simulink model "simu"  (R2023a)
settings: Solver=FixedStepAuto  StartTime=0.0  StopTime=10  RelTol=1e-3
undefined symbols (not defined in the file): Kalpha, Kbeta, Krho, theta_0, x_0, y_0
settings Model: Creator=daneydem1u  LastModifiedBy=daneydem1u

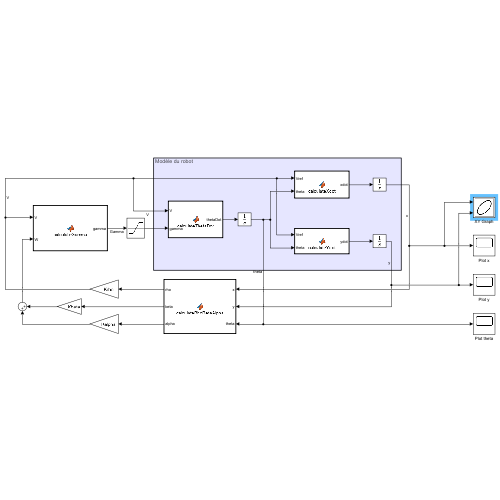
[thumbnail: Simulink's stored preview of the top-level diagram]
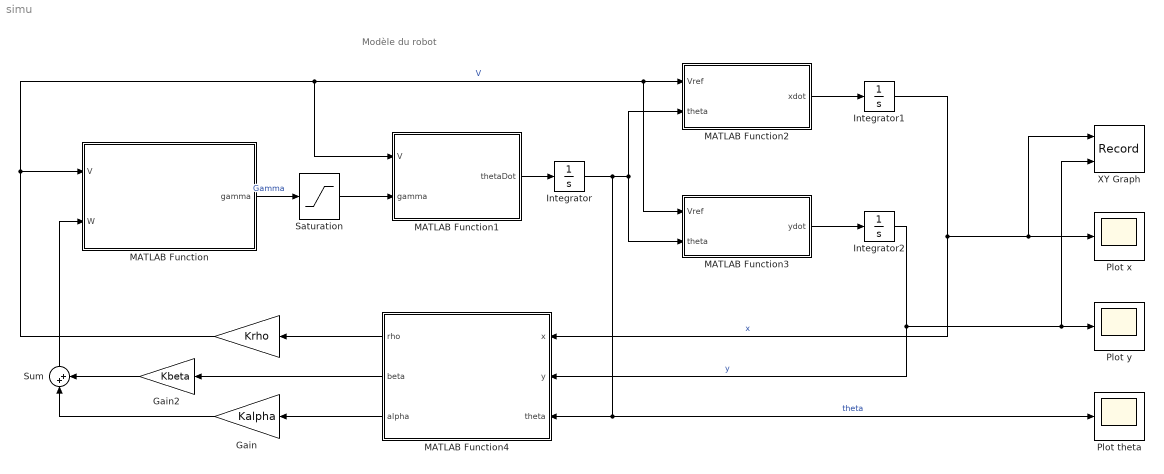
== system simu ==
  note: Modèle du robot
  " " : Gain  Gain=Krho
  Gain : Gain  Gain=Kalpha
  Gain2 : Gain  Gain=Kbeta
  Integrator : Integrator  InitialCondition=theta_0
  Integrator1 : Integrator  InitialCondition=x_0
  Integrator2 : Integrator  InitialCondition=y_0
  MATLAB Function : MATLAB Function  TreatAsAtomicUnit=on
  MATLAB Function1 : MATLAB Function  TreatAsAtomicUnit=on
  MATLAB Function2 : MATLAB Function  TreatAsAtomicUnit=on
  MATLAB Function3 : MATLAB Function  TreatAsAtomicUnit=on
  MATLAB Function4 : MATLAB Function  TreatAsAtomicUnit=on
  Plot theta : Scope
  Plot x : Scope
  Plot y : Scope
  Saturation : Saturate  UpperLimit=pi/2  LowerLimit=-pi/2
  Sum : Sum  Inputs=|++
  XY Graph : Record  FileSettingsInternal="{\"entries\":[{\"content\":{\"excelSettings\":{\"content\":{},\"type\":\"Streamout.ExcelSettings\"}},\"type\":\"Streamout.FileSettingStorage\",\"uuid\":\"87b38950-ab84-4d4e-b85e-4042bda6b861\"}],\"packageUris\":[\"http://schema.mathworks.com/mf0/streamout_blocks/R2020a\"],\"version\":\"1.0\"}"  Layout=[1 1]  SignalsInternal="{\"entries\":[{\"content\":{\"signals\":[{\"content\":{\"blockPath\":[\"simu/XY Graph\"],\"dimensions\":[1],\"domain\":\"simu/XY Graph\",\"lineColor\":\"#a2142f\",\"plots\":[1],\"port\":1,\"sid\":[\"\"],\"signalID\":212,\"signalName\":\"x\"},\"type\":\"RecordBlkView.Signal\",\"uuid\":\"13bd241f-c241-453c-ad47-541923f631b6\"},{\"content\":{\"blockPath\":[\"simu/XY Graph\"],\"dimensions\":[1],\"domain\":\"simu/XY Graph\",\"lineColor\":\"#139fff\",\"plots\":[1],\"port\":2,\"sid\":[\"\"],\"signalID\":216,\"signalName\":\"y\"},\"type\":\"RecordBlkView.Signal\",\"uuid\":\"333290c1-e4d1-4cdb-b6ca-dd34188088a4\"}]},\"type\":\"RecordBlkView.InputSignals\",\"uuid\":\"5faa1cd1-91aa-435c-92d6-fa03ea82110c\"}],\"packageUris\":[\"http://schema.mathworks.com/mf0/streamout_blocks/R2020a\"],\"version\":\"1.0\"}"  VisualizationBindings="{\"xyplotplugin\":{\"info\":[{\"series\":[{\"bindingParametersList\":[{\"parameter\":\"X-Axis\",\"signalID\":212,\"signalName\":\"x\"},{\"parameter\":\"Y-Axis\",\"signalID\":216,\"signalName\":\"y\"}],\"seriesID\":8097}],\"subplotID\":1}]}}"  CompatibilityTag=XY
  wires:
  " "/1 -> MATLAB Function/1(V), MATLAB Function1/1(V), MATLAB Function3/1(Vref), MATLAB Function2/1(Vref)  "V"
  Sum/1 -> MATLAB Function/2(W)
  MATLAB Function1/1(thetaDot) -> Integrator/1
  Integrator/1 -> MATLAB Function4/3(theta), Plot theta/1, MATLAB Function2/2(theta), MATLAB Function3/2(theta)  "theta"
  MATLAB Function2/1(xdot) -> Integrator1/1
  MATLAB Function3/1(ydot) -> Integrator2/1
  Integrator1/1 -> MATLAB Function4/1(x), XY Graph/1, Plot x/1  "x"
  Integrator2/1 -> MATLAB Function4/2(y), XY Graph/2, Plot y/1  "y"
  MATLAB Function4/1(rho) -> " "/1
  MATLAB Function4/2(beta) -> Gain2/1
  MATLAB Function4/3(alpha) -> Gain/1
  Gain2/1 -> Sum/2
  Gain/1 -> Sum/1
  Saturation/1 -> MATLAB Function1/2(gamma)
  MATLAB Function/1(gamma) -> Saturation/1  "Gamma"

== matlab function simu/MATLAB Function1 ==
  data: V input; thetaDot output; gamma input; longueur parameter
function thetaDot = calculateThetaDot(V, gamma, longueur)
    % Calcul de thetaDot
    thetaDot = V * tan(gamma) / longueur;
end

== matlab function simu/MATLAB Function ==
  data: V input; gamma output; W input; longueur parameter
function gamma = calculateGamma(V, W, longueur)
    gamma = atan((W * longueur) / V);
end

== matlab function simu/MATLAB Function2 ==
  data: Vref input; xdot output; theta input
function xdot = calculateXdot(Vref, theta)
    xdot = Vref * cos(theta);
end

== matlab function simu/MATLAB Function3 ==
  data: Vref input; ydot output; theta input
function ydot = calculateYdot(Vref, theta)
    ydot = Vref * sin(theta);
end

== matlab function simu/MATLAB Function4 ==
  data: x input; rho output; y input; theta input; beta output; alpha output
function [rho, beta, alpha] = calculateRhoBetaAlpha(x, y, theta)
    rho = sqrt(x^2 + y^2); % Distance euclidienne à l'origine

    % Calcul de l'angle alpha
    alpha_to_origin = atan2(-y, -x); % Angle entre la position actuelle et l'origine
    alpha = wrapToPi(alpha_to_origin - theta); % Différence d'angle

    % Calcul de l'angle beta
    beta = -theta; % Angle par rapport à l'orientation finale souhaitée (alignée avec l'axe des abscisses)
end
